simulink model "simulinkLAB2"  (R2022b)
settings: Solver=VariableStepAuto  StartTime=0.0  StopTime=10.0  RelTol=1e-3
values from neighbouring files (symbols this model uses):
  J = i^2*Jed    (= 0.002437632)    [ML_lab2_final.m]
  k_e = (k_e_n + k_e_p)/2    [ML_lab2_final.m]
  k_m = k_e    [ML_lab2_final.m]
  L = 0.0047    [ML_lab2_final.m]
  R = (resistance_n + resistance_p)/2    [ML_lab2_final.m]
  U = voltage_n(i)    [ML_lab2_final.m]
settings Model: Creator=user  LastModifiedBy=nkggu

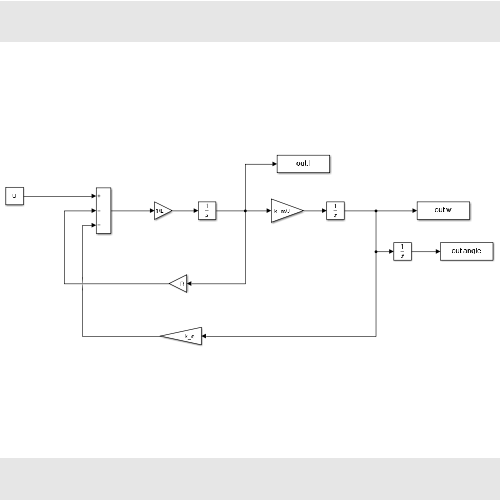
[thumbnail: Simulink's stored preview of the top-level diagram]
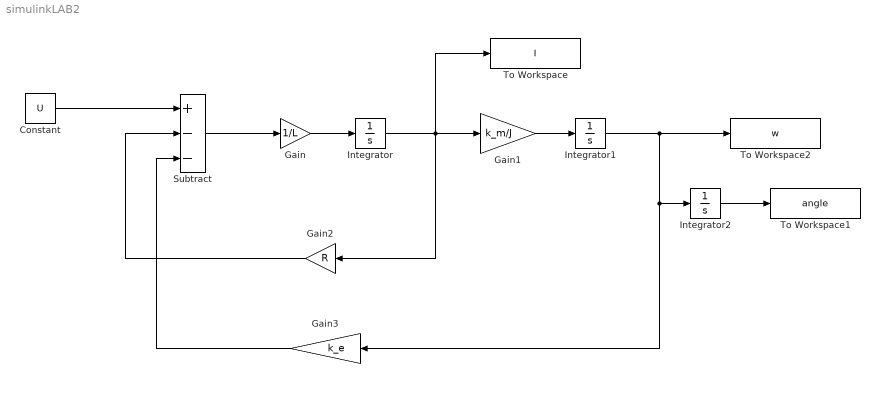
== system simulinkLAB2 ==
  Constant : Constant  Value=U
  Gain : Gain  Gain=1/L
  Gain1 : Gain  Gain=k_m/J
  Gain2 : Gain  Gain=R
  Gain3 : Gain  Gain=k_e
  Integrator : Integrator
  Integrator1 : Integrator
  Integrator2 : Integrator
  Subtract : Sum  Inputs=+--
  To Workspace : ToWorkspace  VariableName=I  SaveFormat=Timeseries  SampleTime=-1
  To Workspace1 : ToWorkspace  VariableName=angle  SaveFormat=Timeseries  SampleTime=-1
  To Workspace2 : ToWorkspace  VariableName=w  SaveFormat=Timeseries  SampleTime=-1
  wires:
  Gain/1 -> Integrator/1
  Integrator/1 -> Gain2/1, Gain1/1, To Workspace/1
  Subtract/1 -> Gain/1
  Gain1/1 -> Integrator1/1
  Gain2/1 -> Subtract/2
  Constant/1 -> Subtract/1
  Integrator1/1 -> To Workspace2/1, Integrator2/1, Gain3/1
  Gain3/1 -> Subtract/3
  Integrator2/1 -> To Workspace1/1
